simulink model "SkywalkerX8_StateEstimation"  (R2018a)
settings: Solver=FixedStepAuto  StartTime=0.0  StopTime=120  FixedStep=0.001  RelTol=1e-3
undefined symbols (not defined in the file): magnitude, SkywalkerX8
libraries: simulink_extras x10, sensors x7, sharedTrackingLibrary x2, dspmtrx3 x1
settings Model: Creator=David  LastModifiedBy=David

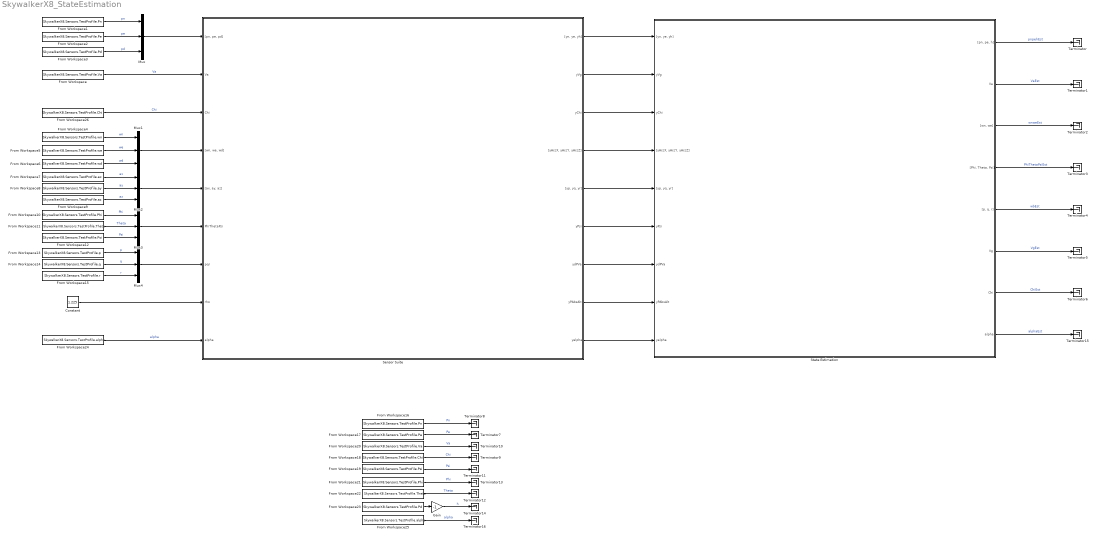
== system SkywalkerX8_StateEstimation ==
  Constant : Constant  Value=1.225
  From Workspace : FromWorkspace  VariableName=SkywalkerX8.Sensors.TestProfile.Va  SampleTime=SkywalkerX8.Sensors.TestProfile.Time(2)  Interpolate=off  OutputAfterFinalValue=Holding final value
  From Workspace1 : FromWorkspace  VariableName=SkywalkerX8.Sensors.TestProfile.Pn  SampleTime=SkywalkerX8.Sensors.TestProfile.Time(2)  Interpolate=off  OutputAfterFinalValue=Holding final value
  From Workspace10 : FromWorkspace  VariableName=SkywalkerX8.Sensors.TestProfile.Phi  SampleTime=SkywalkerX8.Sensors.TestProfile.Time(2)  Interpolate=off  OutputAfterFinalValue=Holding final value
  From Workspace11 : FromWorkspace  VariableName=SkywalkerX8.Sensors.TestProfile.Theta  SampleTime=SkywalkerX8.Sensors.TestProfile.Time(2)  Interpolate=off  OutputAfterFinalValue=Holding final value
  From Workspace12 : FromWorkspace  VariableName=SkywalkerX8.Sensors.TestProfile.Psi  SampleTime=SkywalkerX8.Sensors.TestProfile.Time(2)  Interpolate=off  OutputAfterFinalValue=Holding final value
  From Workspace13 : FromWorkspace  VariableName=SkywalkerX8.Sensors.TestProfile.p  SampleTime=SkywalkerX8.Sensors.TestProfile.Time(2)  Interpolate=off  OutputAfterFinalValue=Holding final value
  From Workspace14 : FromWorkspace  VariableName=SkywalkerX8.Sensors.TestProfile.q  SampleTime=SkywalkerX8.Sensors.TestProfile.Time(2)  Interpolate=off  OutputAfterFinalValue=Holding final value
  From Workspace15 : FromWorkspace  VariableName=SkywalkerX8.Sensors.TestProfile.r  SampleTime=SkywalkerX8.Sensors.TestProfile.Time(2)  Interpolate=off  OutputAfterFinalValue=Holding final value
  From Workspace16 : FromWorkspace  VariableName=SkywalkerX8.Sensors.TestProfile.Pn  Interpolate=off  OutputAfterFinalValue=Holding final value
  From Workspace17 : FromWorkspace  VariableName=SkywalkerX8.Sensors.TestProfile.Pe  Interpolate=off  OutputAfterFinalValue=Holding final value
  From Workspace18 : FromWorkspace  VariableName=SkywalkerX8.Sensors.TestProfile.Chi  Interpolate=off  OutputAfterFinalValue=Holding final value
  From Workspace19 : FromWorkspace  VariableName=SkywalkerX8.Sensors.TestProfile.Psi  Interpolate=off  OutputAfterFinalValue=Holding final value
  From Workspace2 : FromWorkspace  VariableName=SkywalkerX8.Sensors.TestProfile.Pe  SampleTime=SkywalkerX8.Sensors.TestProfile.Time(2)  Interpolate=off  OutputAfterFinalValue=Holding final value
  From Workspace20 : FromWorkspace  VariableName=SkywalkerX8.Sensors.TestProfile.Va  Interpolate=off  OutputAfterFinalValue=Holding final value
  From Workspace21 : FromWorkspace  VariableName=SkywalkerX8.Sensors.TestProfile.Phi  Interpolate=off  OutputAfterFinalValue=Holding final value
  From Workspace22 : FromWorkspace  VariableName=SkywalkerX8.Sensors.TestProfile.Theta  Interpolate=off  OutputAfterFinalValue=Holding final value
  From Workspace23 : FromWorkspace  VariableName=SkywalkerX8.Sensors.TestProfile.Pd  SampleTime=SkywalkerX8.Sensors.TestProfile.Time(2)  Interpolate=off  OutputAfterFinalValue=Holding final value
  From Workspace24 : FromWorkspace  VariableName=SkywalkerX8.Sensors.TestProfile.alpha  SampleTime=SkywalkerX8.Sensors.TestProfile.Time(2)  Interpolate=off  OutputAfterFinalValue=Holding final value
  From Workspace25 : FromWorkspace  VariableName=SkywalkerX8.Sensors.TestProfile.alpha  SampleTime=SkywalkerX8.Sensors.TestProfile.Time(2)  Interpolate=off  OutputAfterFinalValue=Holding final value
  From Workspace26 : FromWorkspace  VariableName=SkywalkerX8.Sensors.TestProfile.Chi  SampleTime=SkywalkerX8.Sensors.TestProfile.Time(2)  Interpolate=off  OutputAfterFinalValue=Holding final value
  From Workspace3 : FromWorkspace  VariableName=SkywalkerX8.Sensors.TestProfile.Pd  SampleTime=SkywalkerX8.Sensors.TestProfile.Time(2)  Interpolate=off  OutputAfterFinalValue=Holding final value
  From Workspace4 : FromWorkspace  VariableName=SkywalkerX8.Sensors.TestProfile.wn  SampleTime=SkywalkerX8.Sensors.TestProfile.Time(2)  Interpolate=off  OutputAfterFinalValue=Holding final value
  From Workspace5 : FromWorkspace  VariableName=SkywalkerX8.Sensors.TestProfile.we  SampleTime=SkywalkerX8.Sensors.TestProfile.Time(2)  Interpolate=off  OutputAfterFinalValue=Holding final value
  From Workspace6 : FromWorkspace  VariableName=SkywalkerX8.Sensors.TestProfile.wd  SampleTime=SkywalkerX8.Sensors.TestProfile.Time(2)  Interpolate=off  OutputAfterFinalValue=Holding final value
  From Workspace7 : FromWorkspace  VariableName=SkywalkerX8.Sensors.TestProfile.ax  SampleTime=SkywalkerX8.Sensors.TestProfile.Time(2)  Interpolate=off  OutputAfterFinalValue=Holding final value
  From Workspace8 : FromWorkspace  VariableName=SkywalkerX8.Sensors.TestProfile.ay  SampleTime=SkywalkerX8.Sensors.TestProfile.Time(2)  Interpolate=off  OutputAfterFinalValue=Holding final value
  From Workspace9 : FromWorkspace  VariableName=SkywalkerX8.Sensors.TestProfile.az  SampleTime=SkywalkerX8.Sensors.TestProfile.Time(2)  Interpolate=off  OutputAfterFinalValue=Holding final value
  Gain : Gain  Gain=-1
  Mux{,1..4} (5 alike) : Mux  Inputs=3
  Sensor Suite : Subsystem
      mask Display:
      | image('telemetry.jpg')
      | 
      | color('cyan')
      | 
      | port_label('input', 1, '[p_N, p_E, p_D] (m)', 'texMode', 'On')
      | port_label('input', 2, 'V_a (m/s)', 'texMode', 'On')
      | port_label('input', 3, '\chi (rad)', 'texMode', 'On')
      | port_label('input', 4, '[w_N, w_E, w_D] (m/s)', 'texMode', 'On')
      | port_label('input', 5, '{\bfa_{inertial}} (m/s^2)', 'texMode', 'on')
      | port_label('input', 6, '[\phi, \theta, \psi] (rad)', 'texMode', 'on')
      | port_label('input', 7, '{\bf\omega_b} (rad/s)', 'texMode', 'on')
      | port_label('input', 8, '\rho (kg/m^3)', 'texMode', 'on')
      | port_label('input', 9, '\alpha (rad)', 'texMode', 'on')
      | 
      | port_label('output', 1, '[y_{GPS_N}, y_{GPS_E}, y_{GPS_h}] (m)', 'texMode', 'On')
      | port_label('output', 2, 'y_{GPS_{Vg}} (m/s)', 'texMode', 'On')
      | port_label('output', 3, 'y_{GPS_{\chi}} (rad)', 'texMode', 'On')
      | port_label('output', 4, '[y_{accel_x}, y_{accel_y}, y_{accel_z}] (m/s^2)', 'texMode', 'on')
      | port_label('output', 5, '[y_p, y_q, y_r] (rad/s)', 'texMode', 'on')
      | port_label('output', 6, 'y_{\psi} (rad)', 'texMode', 'on')
      | port_label('output', 7, 'y_{\DeltaP_{V_a}} (Pa)', 'texMode', 'on')
      | port_label('output', 8, 'y_{P_{abs}} (Pa)', 'texMode', 'on')
      | port_label('output', 9, 'y_\alpha (rad)', 'texMode', 'on')
  State Estimation : Subsystem
      mask Display:
      | image('state_estimate.jpg', 'center')
      | 
      | port_label('input', 1, '[y_{GPS_N}, y_{GPS_E}, y_{GPS_h}] (m)', 'texMode', 'On')
      | port_label('input', 2, 'y_{GPS_{Vg}} (m/s)', 'texMode', 'On')
      | port_label('input', 3, 'y_{GPS_{\chi}} (rad)', 'texMode', 'On')
      | port_label('input', 4, '[y_{accel_x}, y_{accel_y}, y_{accel_z}] (m/s^2)', 'texMode', 'on')
      | port_label('input', 5, '[y_p, y_q, y_r] (rad/s)', 'texMode', 'on')
      | port_label('input', 6, 'y_{\psi} (rad)', 'texMode', 'on')
      | port_label('input', 7, 'y_{\DeltaP_{V_a}} (Pa)', 'texMode', 'on')
      | port_label('input', 8, 'y_{P_{abs}} (Pa)', 'texMode', 'on')
      | port_label('input', 9, 'y_{\alpha} (rad)', 'texMode', 'on')
      | 
      | port_label('output', 1, '[p_N, p_E, h] (m)', 'texMode', 'On')
      | port_label('output', 2, 'V_a (m/s)', 'texMode', 'On')
      | port_label('output', 3, '[w_N, w_E] (m/s)', 'texMode', 'On')
      | port_label('output', 4, '[\phi, \theta, \psi] (rad)', 'texMode', 'on')
      | port_label('output', 5, '{\bf\omega_b} (rad/s)', 'texMode', 'on')
      | port_label('output', 6, 'V_g (m/s)', 'texMode', 'on')
      | port_label('output', 7, '\chi (rad)', 'texMode', 'on')
      | port_label('output', 8, '\alpha (rad)', 'texMode', 'on')
  Terminator{,1..16} (17 alike) : Terminator
  wires:
  Mux2/1 -> Sensor Suite/5("[ax, ay, az]")
  From Workspace14/1 -> Mux4/2  "q"
  From Workspace2/1 -> Mux/2  "pe"
  From Workspace10/1 -> Mux3/1  "Phi"
  Mux1/1 -> Sensor Suite/4("[wn, we, wd]")
  From Workspace13/1 -> Mux4/1  "p"
  From Workspace1/1 -> Mux/1  "pn"
  Constant/1 -> Sensor Suite/8(rho)
  From Workspace11/1 -> Mux3/2  "Theta"
  From Workspace4/1 -> Mux1/1  "wn"
  From Workspace7/1 -> Mux2/1  "ax"
  From Workspace6/1 -> Mux1/3  "wd"
  From Workspace9/1 -> Mux2/3  "az"
  From Workspace12/1 -> Mux3/3  "Psi"
  From Workspace/1 -> Sensor Suite/2(Va)  "Va"
  From Workspace3/1 -> Mux/3  "pd"
  Mux4/1 -> Sensor Suite/7(pqr)
  From Workspace8/1 -> Mux2/2  "ay"
  Mux3/1 -> Sensor Suite/6(PhiThetaPsi)
  From Workspace5/1 -> Mux1/2  "we"
  From Workspace15/1 -> Mux4/3  "r"
  Mux/1 -> Sensor Suite/1("[pn, pe, pd]")
  State Estimation/1("[pn, pe, h]") -> Terminator/1  "pnpehEst"
  State Estimation/2(Va) -> Terminator1/1  "VaEst"
  State Estimation/3("[wn, we]") -> Terminator2/1  "wnweEst"
  State Estimation/4("[Phi, Theta, Psi]") -> Terminator3/1  "PhiThetaPsiEst"
  State Estimation/5("[p, q, r]") -> Terminator4/1  "wbEst"
  State Estimation/6(Vg) -> Terminator5/1  "VgEst"
  State Estimation/7(Chi) -> Terminator6/1  "ChiEst"
  From Workspace20/1 -> Terminator10/1  "Va"
  From Workspace16/1 -> Terminator8/1  "Pn"
  From Workspace18/1 -> Terminator9/1  "Chi"
  From Workspace19/1 -> Terminator11/1  "Psi"
  From Workspace17/1 -> Terminator7/1  "Pe"
  From Workspace21/1 -> Terminator13/1  "Phi"
  From Workspace22/1 -> Terminator12/1  "Theta"
  From Workspace23/1 -> Gain/1
  Gain/1 -> Terminator14/1  "h"
  Sensor Suite/9(yalpha) -> State Estimation/9(yalpha)
  Sensor Suite/8(yPAbsAlt) -> State Estimation/8(yPAbsAlt)
  Sensor Suite/7(ydPVa) -> State Estimation/7(ydPVa)
  Sensor Suite/6(yPsi) -> State Estimation/6(yPsi)
  Sensor Suite/5("[yp, yq, yr]") -> State Estimation/5("[yp, yq, yr]")
  Sensor Suite/4("[yAccX, yAccY, yAccZ]") -> State Estimation/4("[yAccX, yAccY, yAccZ]")
  Sensor Suite/3(yChi) -> State Estimation/3(yChi)
  Sensor Suite/2(yVg) -> State Estimation/2(yVg)
  Sensor Suite/1("[yn, ye, yh]") -> State Estimation/1("[yn, ye, yh]")
  State Estimation/8(alpha) -> Terminator15/1  "alphaEst"
  From Workspace24/1 -> Sensor Suite/9(alpha)  "alpha"
  From Workspace25/1 -> Terminator16/1  "alpha"
  From Workspace26/1 -> Sensor Suite/3(Chi)  "Chi"

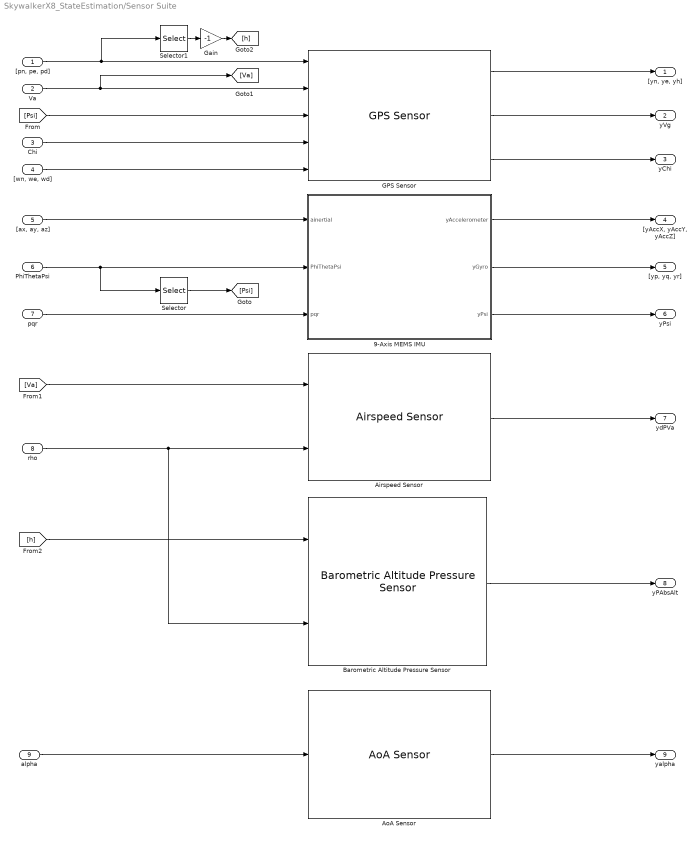
== system SkywalkerX8_StateEstimation/Sensor Suite ==
  "[pn, pe, pd]" : Inport
  Va : Inport  Port=2
  Chi : Inport  Port=3
  "[wn, we, wd]" : Inport  Port=4
  "[ax, ay, az]" : Inport  Port=5
  PhiThetaPsi : Inport  Port=6
  pqr : Inport  Port=7
  rho : Inport  Port=8
  alpha : Inport  Port=9
  9-Axis MEMS IMU : Subsystem
      mask Display:
      | image('VNAV_IMU.jpg')
      | 
      | color('green')
      | 
      | port_label('input', 1, '{\bfa_{inertial}} (m/s^2)', 'texMode', 'on')
      | port_label('input', 2, '[\phi, \theta, \psi] (rad)', 'texMode', 'on')
      | port_label('input', 3, '{\bf\omega_b} (rad/s)', 'texMode', 'on')
      | 
      | port_label('output', 1, '[y_{accel_x}, y_{accel_y}, y_{accel_z}] (m/s^2)', 'texMode', 'on')
      | port_label('output', 2, '[y_p, y_q, y_r] (rad/s)', 'texMode', 'on')
      | port_label('output', 3, 'y_{\psi} (rad)', 'texMode', 'on')
  Airspeed Sensor : sensors/Airspeed Sensor  SampleTime=SkywalkerX8.Sensors.AirspeedPressure.SampleTime  diffPressureStdDev=SkywalkerX8.Sensors.AirspeedPressure.StdDev  diffPressureBandwidthHz=SkywalkerX8.Sensors.AirspeedPressure.BandwidthHz  diffPressureInit=SkywalkerX8.Sensors.AirspeedPressure.InitialCondition  diffPressureUpperSaturation=SkywalkerX8.Sensors.AirspeedPressure.UpperSat  diffPressureLowerSaturation=SkywalkerX8.Sensors.AirspeedPressure.LowerSat  diffPressureResolution=SkywalkerX8.Sensors.AirspeedPressure.Resolution
  AoA Sensor : sensors/AoA Sensor  SampleTime=SkywalkerX8.Sensors.AoA.SampleTime  alphaStdDev=SkywalkerX8.Sensors.AoA.StdDev  alphaBandwidthHz=SkywalkerX8.Sensors.AoA.BandwidthHz  alphaInit=SkywalkerX8.Sensors.AoA.InitialCondition  alphaUpperSaturation=SkywalkerX8.Sensors.AoA.UpperSat  alphaLowerSaturation=SkywalkerX8.Sensors.AoA.LowerSat  alphaResolution=SkywalkerX8.Sensors.AoA.Resolution
  Barometric Altitude Pressure Sensor : sensors/Barometric Altitude Pressure Sensor  g=SkywalkerX8.System.Gravity  SampleTime=SkywalkerX8.Sensors.AltitudePressure.SampleTime  absPressureStdDev=SkywalkerX8.Sensors.AltitudePressure.StdDev  absPressureBandwidthHz=SkywalkerX8.Sensors.AltitudePressure.BandwidthHz  absPressureInit=SkywalkerX8.Sensors.AltitudePressure.InitialCondition  absPressureUpperSaturation=SkywalkerX8.Sensors.AltitudePressure.UpperSat  absPressureLowerSaturation=SkywalkerX8.Sensors.AltitudePressure.LowerSat  absPressureResolution=SkywalkerX8.Sensors.AltitudePressure.Resolution
  GPS Sensor : sensors/GPS Sensor  SampleTime=SkywalkerX8.Sensors.GPS.SampleTime  pnInit=SkywalkerX8.Sensors.GPS.pnInit  peInit=SkywalkerX8.Sensors.GPS.peInit  pdInit=SkywalkerX8.Sensors.GPS.pdInit  VgInit=SkywalkerX8.Sensors.GPS.VgInit  ChiInit=SkywalkerX8.Sensors.GPS.ChiInit  GPSNStdDev=SkywalkerX8.Sensors.GPS.North.StdDev  OneOverkGPSN=SkywalkerX8.Sensors.GPS.North.TimeConstant  GPSEStdDev=SkywalkerX8.Sensors.GPS.East.StdDev  OneOverkGPSE=SkywalkerX8.Sensors.GPS.East.TimeConstant  GPSAltStdDev=SkywalkerX8.Sensors.GPS.Alt.StdDev  OneOverkGPSAlt=SkywalkerX8.Sensors.GPS.Alt.TimeConstant  GPSVStdDev=SkywalkerX8.Sensors.GPS.Velocity.StdDev
  Gain : Gain  Gain=-1
  Selector : Selector  InputPortWidth=3  IndexOptions=Index vector (dialog)  Indices=3  OutputSizes=1
  Selector1 : Selector  InputPortWidth=3  IndexOptions=Index vector (dialog)  Indices=3  OutputSizes=1
  "[yn, ye, yh]" : Outport
  yVg : Outport  Port=2
  yChi : Outport  Port=3
  "[yAccX, yAccY, yAccZ]" : Outport  Port=4
  "[yp, yq, yr]" : Outport  Port=5
  yPsi : Outport  Port=6
  ydPVa : Outport  Port=7
  yPAbsAlt : Outport  Port=8
  yalpha : Outport  Port=9
  wires:
  "[pn, pe, pd]"/1 -> GPS Sensor/1, Selector1/1
  Va/1 -> GPS Sensor/2, [Va]
  PhiThetaPsi/1 -> 9-Axis MEMS IMU/2(PhiThetaPsi), Selector/1
  Airspeed Sensor/1 -> ydPVa/1
  [Psi] -> GPS Sensor/3
  Selector1/1 -> Gain/1
  rho/1 -> Barometric Altitude Pressure Sensor/2, Airspeed Sensor/2
  GPS Sensor/3 -> yChi/1
  Selector/1 -> [Psi]
  [h] -> Barometric Altitude Pressure Sensor/1
  9-Axis MEMS IMU/3(yPsi) -> yPsi/1
  [Va] -> Airspeed Sensor/1
  pqr/1 -> 9-Axis MEMS IMU/3(pqr)
  9-Axis MEMS IMU/2(yGyro) -> "[yp, yq, yr]"/1
  "[wn, we, wd]"/1 -> GPS Sensor/5
  Barometric Altitude Pressure Sensor/1 -> yPAbsAlt/1
  GPS Sensor/1 -> "[yn, ye, yh]"/1
  Gain/1 -> [h]
  GPS Sensor/2 -> yVg/1
  "[ax, ay, az]"/1 -> 9-Axis MEMS IMU/1(ainertial)
  9-Axis MEMS IMU/1(yAccelerometer) -> "[yAccX, yAccY, yAccZ]"/1
  AoA Sensor/1 -> yalpha/1
  alpha/1 -> AoA Sensor/1
  Chi/1 -> GPS Sensor/4

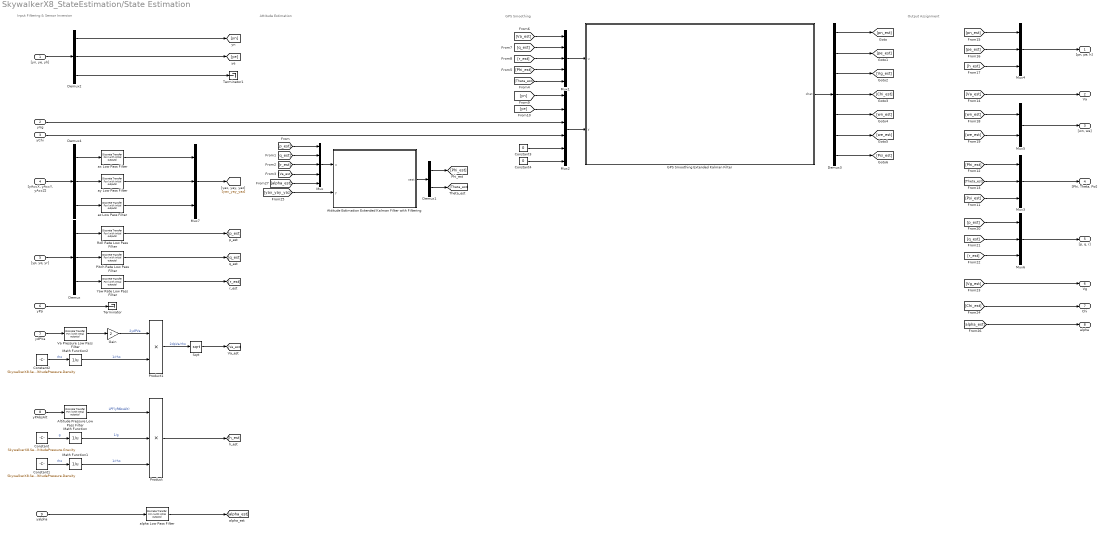
== system SkywalkerX8_StateEstimation/State Estimation ==
  note: Output Assignment
  note: GPS Smoothing
  note: Attitude Estimation
  note: Input Filtering & Sensor Inversion
  "[yn, ye, yh]" : Inport  PortDimensions=3
  yVg : Inport  Port=2
  yChi : Inport  Port=3
  "[yAccX, yAccY, yAccZ]" : Inport  Port=4  PortDimensions=3
  "[yp, yq, yr]" : Inport  Port=5  PortDimensions=3
  yPsi : Inport  Port=6
  ydPVa : Inport  Port=7
  yPAbsAlt : Inport  Port=8
  yalpha : Inport  Port=9
  Altitude Pressure Low Pass Filter : simulink_extras/Additional Discrete/Discrete Transfer Fcn (with initial outputs)  N=cell2mat(SkywalkerX8.Sensors.Filters.AltitudePressure.FilterTFDigital.Numerator)  D=cell2mat(SkywalkerX8.Sensors.Filters.AltitudePressure.FilterTFDigital.Denominator)  U0=SkywalkerX8.Sensors.Filters.AltitudePressure.InitialCondition  Y0=SkywalkerX8.Sensors.Filters.AltitudePressure.InitialCondition  TS=SkywalkerX8.Sensors.Filters.AltitudePressure.FilterSampleTime
      settings: SourceProductName=Simulink  SourceProductBaseCode=SL
  Attitude Estimation Extended Kalman Filter with Filtering : Subsystem
      mask Display:
      | port_label('input', 1, '{\bf u} = [p, q, r, V_a, \alpha]', 'texMode', 'On')
      | port_label('input', 2, '{\bf y} = [a_x, a_y, a_z]', 'texMode', 'On')
      | 
      | port_label('output', 1, '{\bf x_{est}} = [\Phi, \theta]', 'texMode', 'On')
  Constant : Constant  Value=SkywalkerX8.Sensors.StateEstimate.SensorInversion.AltitudePressure.Gravity
  Constant1 : Constant  Value=SkywalkerX8.Sensors.StateEstimate.SensorInversion.AltitudePressure.Density
  Constant2 : Constant  Value=SkywalkerX8.Sensors.StateEstimate.SensorInversion.AltitudePressure.Density
  Constant3 : Constant  Value=0
  Constant4 : Constant  Value=0
  Demux : Demux  Outputs=3
  Demux1 : Demux  Outputs=2
  Demux2 : Demux  Outputs=3
  Demux3 : Demux  Outputs=7
  Demux4 : Demux  Outputs=3
  GPS Smoothing Extended Kalman Filter : Subsystem
      mask Display:
      | port_label('input', 1, '{\bf u} = [V_a, q, r, \Phi, \theta]', 'texMode', 'On')
      | port_label('input', 2, '{\bf y} = [y_{GPS_N}, y_{GPS_E}, y_{GPS_{V_g}}, y_{GPS_\chi}, y_{GPS_{wind_N}}, y_{GPS_{wind_E}}]', 'texMode', 'On')
      | 
      | port_label('output', 1, '{\bf x_{est}} = [p_n, p_e, V_g, \chi, w_n, w_e, \psi]', 'texMode', 'On')
  Gain : Gain  Gain=2
  Math Function : Math  Operator=reciprocal  SaturateOnIntegerOverflow=on
  Math Function1 : Math  Operator=reciprocal  SaturateOnIntegerOverflow=on
  Math Function2 : Math  Operator=reciprocal  SaturateOnIntegerOverflow=on
  Mux : Mux  Inputs=5
  Mux1 : Mux  Inputs=5
  Mux2 : Mux  Inputs=6
  Mux{3..4,6..7} (4 alike) : Mux  Inputs=3
  Mux5 : Mux  Inputs=2
  Pitch Rate Low Pass Filter : simulink_extras/Additional Discrete/Discrete Transfer Fcn (with initial outputs)  N=cell2mat(SkywalkerX8.Sensors.Filters.AngularRates.Pitch.FilterTFDigital.Numerator)  D=cell2mat(SkywalkerX8.Sensors.Filters.AngularRates.Pitch.FilterTFDigital.Denominator)  U0=SkywalkerX8.Sensors.Filters.AngularRates.Pitch.InitialCondition  Y0=SkywalkerX8.Sensors.Filters.AngularRates.Pitch.InitialCondition  TS=SkywalkerX8.Sensors.Filters.AngularRates.Pitch.FilterSampleTime
      settings: SourceProductName=Simulink  SourceProductBaseCode=SL
  Product : Product  Inputs=3
  Product1 : Product
  Roll Rate Low Pass Filter : simulink_extras/Additional Discrete/Discrete Transfer Fcn (with initial outputs)  N=cell2mat(SkywalkerX8.Sensors.Filters.AngularRates.Roll.FilterTFDigital.Numerator)  D=cell2mat(SkywalkerX8.Sensors.Filters.AngularRates.Roll.FilterTFDigital.Denominator)  U0=SkywalkerX8.Sensors.Filters.AngularRates.Roll.InitialCondition  Y0=SkywalkerX8.Sensors.Filters.AngularRates.Roll.InitialCondition  TS=SkywalkerX8.Sensors.Filters.AngularRates.Roll.FilterSampleTime
      settings: SourceProductName=Simulink  SourceProductBaseCode=SL
  Sqrt : Sqrt  SaturateOnIntegerOverflow=on
  Terminator : Terminator
  Terminator1 : Terminator
  Va Pressure Low Pass Filter : simulink_extras/Additional Discrete/Discrete Transfer Fcn (with initial outputs)  N=cell2mat(SkywalkerX8.Sensors.Filters.AirspeedPressure.FilterTFDigital.Numerator)  D=cell2mat(SkywalkerX8.Sensors.Filters.AirspeedPressure.FilterTFDigital.Denominator)  U0=SkywalkerX8.Sensors.Filters.AirspeedPressure.InitialCondition  Y0=SkywalkerX8.Sensors.Filters.AirspeedPressure.InitialCondition  TS=SkywalkerX8.Sensors.Filters.AirspeedPressure.FilterSampleTime
      settings: SourceProductName=Simulink  SourceProductBaseCode=SL
  Yaw Rate Low Pass Filter : simulink_extras/Additional Discrete/Discrete Transfer Fcn (with initial outputs)  N=cell2mat(SkywalkerX8.Sensors.Filters.AngularRates.Yaw.FilterTFDigital.Numerator)  D=cell2mat(SkywalkerX8.Sensors.Filters.AngularRates.Yaw.FilterTFDigital.Denominator)  U0=SkywalkerX8.Sensors.Filters.AngularRates.Yaw.InitialCondition  Y0=SkywalkerX8.Sensors.Filters.AngularRates.Yaw.InitialCondition  TS=SkywalkerX8.Sensors.Filters.AngularRates.Yaw.FilterSampleTime
      settings: SourceProductName=Simulink  SourceProductBaseCode=SL
  alpha Low Pass Filter : simulink_extras/Additional Discrete/Discrete Transfer Fcn (with initial outputs)  N=cell2mat(SkywalkerX8.Sensors.Filters.AoA.FilterTFDigital.Numerator)  D=cell2mat(SkywalkerX8.Sensors.Filters.AoA.FilterTFDigital.Denominator)  U0=SkywalkerX8.Sensors.Filters.AoA.InitialCondition  Y0=SkywalkerX8.Sensors.Filters.AoA.InitialCondition  TS=SkywalkerX8.Sensors.Filters.AoA.FilterSampleTime
      settings: SourceProductName=Simulink  SourceProductBaseCode=SL
  ax Low Pass Filter : simulink_extras/Additional Discrete/Discrete Transfer Fcn (with initial outputs)  N=cell2mat(SkywalkerX8.Sensors.EKF.Attitude.Filters.axFilterTFDigital.Numerator)  D=cell2mat(SkywalkerX8.Sensors.EKF.Attitude.Filters.axFilterTFDigital.Denominator)  U0=SkywalkerX8.Sensors.EKF.Attitude.InitialMeasurement(1)  Y0=SkywalkerX8.Sensors.EKF.Attitude.InitialMeasurement(1)  TS=SkywalkerX8.Sensors.EKF.Attitude.Filters.aFilterSampleTime
      settings: SourceProductName=Simulink  SourceProductBaseCode=SL
  ay Low Pass Filter : simulink_extras/Additional Discrete/Discrete Transfer Fcn (with initial outputs)  N=cell2mat(SkywalkerX8.Sensors.EKF.Attitude.Filters.ayFilterTFDigital.Numerator)  D=cell2mat(SkywalkerX8.Sensors.EKF.Attitude.Filters.ayFilterTFDigital.Denominator)  U0=SkywalkerX8.Sensors.EKF.Attitude.InitialMeasurement(2)  Y0=SkywalkerX8.Sensors.EKF.Attitude.InitialMeasurement(2)  TS=SkywalkerX8.Sensors.EKF.Attitude.Filters.aFilterSampleTime
      settings: SourceProductName=Simulink  SourceProductBaseCode=SL
  az Low Pass Filter : simulink_extras/Additional Discrete/Discrete Transfer Fcn (with initial outputs)  N=cell2mat(SkywalkerX8.Sensors.EKF.Attitude.Filters.azFilterTFDigital.Numerator)  D=cell2mat(SkywalkerX8.Sensors.EKF.Attitude.Filters.azFilterTFDigital.Denominator)  U0=SkywalkerX8.Sensors.EKF.Attitude.InitialMeasurement(3)  Y0=SkywalkerX8.Sensors.EKF.Attitude.InitialMeasurement(3)  TS=SkywalkerX8.Sensors.EKF.Attitude.Filters.aFilterSampleTime
      settings: SourceProductName=Simulink  SourceProductBaseCode=SL
  "[pn, pe, h]" : Outport
  Va : Outport  Port=2
  "[wn, we]" : Outport  Port=3
  "[Phi, Theta, Psi]" : Outport  Port=4
  "[p, q, r]" : Outport  Port=5
  Vg : Outport  Port=6
  Chi : Outport  Port=7
  alpha : Outport  Port=8
  wires:
  [Phi_est] -> Mux1/4
  Math Function1/1 -> Product/3  "1/rho"
  [ye] -> Mux2/2
  Sqrt/1 -> [Va_est]
  Demux/2 -> Pitch Rate Low Pass Filter/1
  [r_est] -> Mux/3
  Math Function2/1 -> Product1/2  "1/rho"
  yChi/1 -> Mux2/4
  Demux2/3 -> Terminator1/1
  Mux4/1 -> "[pn, pe, h]"/1
  Mux6/1 -> "[p, q, r]"/1
  [r_est] -> Mux1/3
  Constant3/1 -> Mux2/5
  Constant2/1 -> Math Function2/1  "rho"
  Demux3/4 -> [Chi_est]
  Demux3/3 -> [Vg_est]
  [h_est] -> Mux4/3
  Math Function/1 -> Product/2  "1/g"
  [we_est] -> Mux5/2
  "[yp, yq, yr]"/1 -> Demux/1
  [Theta_est] -> Mux1/5
  Demux3/7 -> [Psi_est]
  Mux2/1 -> GPS Smoothing Extended Kalman Filter/2(y)
  Constant4/1 -> Mux2/6
  [r_est] -> Mux6/3
  Mux/1 -> Attitude Estimation Extended Kalman Filter with Filtering/1(u)
  [wn_est] -> Mux5/1
  Demux2/2 -> [ye]
  GPS Smoothing Extended Kalman Filter/1(xhat) -> Demux3/1
  Constant1/1 -> Math Function1/1  "rho"
  Demux2/1 -> [yn]
  Demux3/6 -> [we_est]
  [q_est] -> Mux6/2
  "[yAccX, yAccY, yAccZ]"/1 -> Demux4/1
  Demux1/2 -> [Theta_est]
  Mux1/1 -> GPS Smoothing Extended Kalman Filter/1(u)
  Demux3/5 -> [wn_est]
  Attitude Estimation Extended Kalman Filter with Filtering/1(xest) -> Demux1/1
  Gain/1 -> Product1/1  "2ydPVa"
  Constant/1 -> Math Function/1  "g"
  [p_est] -> Mux/1
  yVg/1 -> Mux2/3
  Altitude Pressure Low Pass Filter/1 -> Product/1  "LPF(yPAbsAlt)"
  [Chi_est] -> Chi/1
  yPsi/1 -> Terminator/1
  [q_est] -> Mux1/2
  Demux3/1 -> [pn_est]
  [Va_est] -> Mux1/1
  [Theta_est] -> Mux3/2
  Va Pressure Low Pass Filter/1 -> Gain/1
  [q_est] -> Mux/2
  Product1/1 -> Sqrt/1  "2dpVa/rho"
  Yaw Rate Low Pass Filter/1 -> [r_est]
  Product/1 -> [h_est]
  [Va_est] -> Mux/4
  ydPVa/1 -> Va Pressure Low Pass Filter/1
  [Psi_est] -> Mux3/3
  Pitch Rate Low Pass Filter/1 -> [q_est]
  Demux/1 -> Roll Rate Low Pass Filter/1
  yPAbsAlt/1 -> Altitude Pressure Low Pass Filter/1
  Demux/3 -> Yaw Rate Low Pass Filter/1
  [pn_est] -> Mux4/1
  [p_est] -> Mux6/1
  Demux3/2 -> [pe_est]
  Demux1/1 -> [Phi_est]
  [Vg_est] -> Vg/1
  "[yn, ye, yh]"/1 -> Demux2/1
  [pe_est] -> Mux4/2
  [Phi_est] -> Mux3/1
  Mux3/1 -> "[Phi, Theta, Psi]"/1
  Mux5/1 -> "[wn, we]"/1
  [Va_est] -> Va/1
  [yn] -> Mux2/1
  Roll Rate Low Pass Filter/1 -> [p_est]
  Demux4/1 -> ax Low Pass Filter/1
  Demux4/2 -> ay Low Pass Filter/1
  Demux4/3 -> az Low Pass Filter/1
  ax Low Pass Filter/1 -> Mux7/1
  ay Low Pass Filter/1 -> Mux7/2
  az Low Pass Filter/1 -> Mux7/3
  Mux7/1 -> [yax_yay_yaz]
  [yax_yay_yaz] -> Attitude Estimation Extended Kalman Filter with Filtering/2(y)
  yalpha/1 -> alpha Low Pass Filter/1
  alpha Low Pass Filter/1 -> [alpha_est]
  [alpha_est] -> alpha/1
  [alpha_est] -> Mux/5

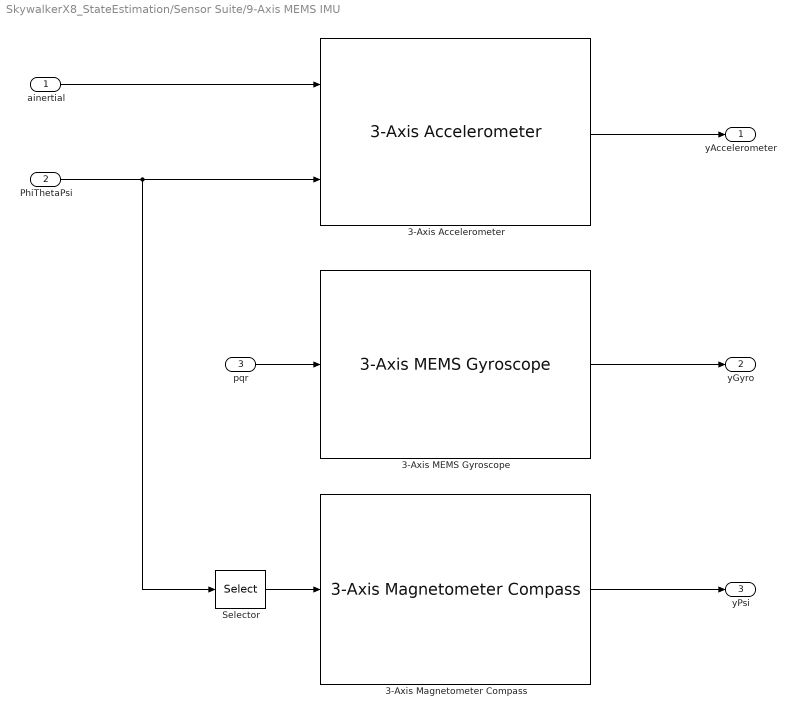
== system SkywalkerX8_StateEstimation/Sensor Suite/9-Axis MEMS IMU ==
  ainertial : Inport
  PhiThetaPsi : Inport  Port=2
  pqr : Inport  Port=3
  3-Axis Accelerometer : sensors/3-Axis Accelerometer  g=SkywalkerX8.System.Gravity  SampleTime=SkywalkerX8.Sensors.IMU.Accelerometer.SampleTime  accelXNoiseDensity=SkywalkerX8.Sensors.IMU.Accelerometer.X.NoiseDensity  accelYNoiseDensity=SkywalkerX8.Sensors.IMU.Accelerometer.Y.NoiseDensity  accelZNoiseDensity=SkywalkerX8.Sensors.IMU.Accelerometer.Z.NoiseDensity  accelXBandwidthHz=SkywalkerX8.Sensors.IMU.Accelerometer.X.BandwidthHz  accelYBandwidthHz=SkywalkerX8.Sensors.IMU.Accelerometer.Y.BandwidthHz  accelZBandwidthHz=SkywalkerX8.Sensors.IMU.Accelerometer.Z.BandwidthHz  accelXInit=SkywalkerX8.Sensors.IMU.Accelerometer.X.InitialCondition  accelYInit=SkywalkerX8.Sensors.IMU.Accelerometer.Y.InitialCondition  accelZInit=SkywalkerX8.Sensors.IMU.Accelerometer.Z.InitialCondition  accelXUpperSaturation=SkywalkerX8.Sensors.IMU.Accelerometer.X.UpperSat  accelXLowerSaturation=SkywalkerX8.Sensors.IMU.Accelerometer.X.LowerSat  accelYUpperSaturation=SkywalkerX8.Sensors.IMU.Accelerometer.Y.UpperSat  accelYLowerSaturation=SkywalkerX8.Sensors.IMU.Accelerometer.Y.LowerSat  accelZUpperSaturation=SkywalkerX8.Sensors.IMU.Accelerometer.Z.UpperSat  accelZLowerSaturation=SkywalkerX8.Sensors.IMU.Accelerometer.Z.LowerSat  accelXResolution=SkywalkerX8.Sensors.IMU.Accelerometer.X.Resolution  accelYResolution=SkywalkerX8.Sensors.IMU.Accelerometer.Y.Resolution  accelZResolution=SkywalkerX8.Sensors.IMU.Accelerometer.Z.Resolution
  3-Axis MEMS Gyroscope : sensors/3-Axis MEMS Gyroscope  SampleTime=SkywalkerX8.Sensors.IMU.Gyroscope.SampleTime  gyroXNoiseDensity=SkywalkerX8.Sensors.IMU.Gyroscope.X.NoiseDensity  gyroYNoiseDensity=SkywalkerX8.Sensors.IMU.Gyroscope.Y.NoiseDensity  gyroZNoiseDensity=SkywalkerX8.Sensors.IMU.Gyroscope.Z.NoiseDensity  gyroXBandwidthHz=SkywalkerX8.Sensors.IMU.Gyroscope.X.BandwidthHz  gyroYBandwidthHz=SkywalkerX8.Sensors.IMU.Gyroscope.Y.BandwidthHz  gyroZBandwidthHz=SkywalkerX8.Sensors.IMU.Gyroscope.Z.BandwidthHz  gyroXInit=SkywalkerX8.Sensors.IMU.Gyroscope.X.InitialCondition  gyroYInit=SkywalkerX8.Sensors.IMU.Gyroscope.Y.InitialCondition  gyroZInit=SkywalkerX8.Sensors.IMU.Gyroscope.Z.InitialCondition  gyroXUpperSaturation=SkywalkerX8.Sensors.IMU.Gyroscope.X.UpperSat  gyroXLowerSaturation=SkywalkerX8.Sensors.IMU.Gyroscope.X.LowerSat  gyroYUpperSaturation=SkywalkerX8.Sensors.IMU.Gyroscope.Y.UpperSat  gyroYLowerSaturation=SkywalkerX8.Sensors.IMU.Gyroscope.Y.LowerSat  gyroZUpperSaturation=SkywalkerX8.Sensors.IMU.Gyroscope.Z.UpperSat  gyroZLowerSaturation=SkywalkerX8.Sensors.IMU.Gyroscope.Z.LowerSat  gyroXResolution=SkywalkerX8.Sensors.IMU.Gyroscope.X.Resolution  gyroYResolution=SkywalkerX8.Sensors.IMU.Gyroscope.Y.Resolution  gyroZResolution=SkywalkerX8.Sensors.IMU.Gyroscope.Z.Resolution
  3-Axis Magnetometer Compass : sensors/3-Axis Magnetometer Compass  SampleTime=SkywalkerX8.Sensors.IMU.Compass.SampleTime  headingNoiseDensity=SkywalkerX8.Sensors.IMU.Compass.NoiseDensity  headingBandwidthHz=SkywalkerX8.Sensors.IMU.Compass.BandwidthHz  headingInit=SkywalkerX8.Sensors.IMU.Compass.InitialCondition  headingUpperSaturation=SkywalkerX8.Sensors.IMU.Compass.UpperSat  headingLowerSaturation=SkywalkerX8.Sensors.IMU.Compass.LowerSat  headingResolution=SkywalkerX8.Sensors.IMU.Compass.Resolution
  Selector : Selector  InputPortWidth=3  IndexOptions=Index vector (dialog)  Indices=3  OutputSizes=1
  yAccelerometer : Outport
  yGyro : Outport  Port=2
  yPsi : Outport  Port=3
  wires:
  ainertial/1 -> 3-Axis Accelerometer/1
  PhiThetaPsi/1 -> 3-Axis Accelerometer/2, Selector/1
  Selector/1 -> 3-Axis Magnetometer Compass/1
  pqr/1 -> 3-Axis MEMS Gyroscope/1
  3-Axis MEMS Gyroscope/1 -> yGyro/1
  3-Axis Accelerometer/1 -> yAccelerometer/1
  3-Axis Magnetometer Compass/1 -> yPsi/1

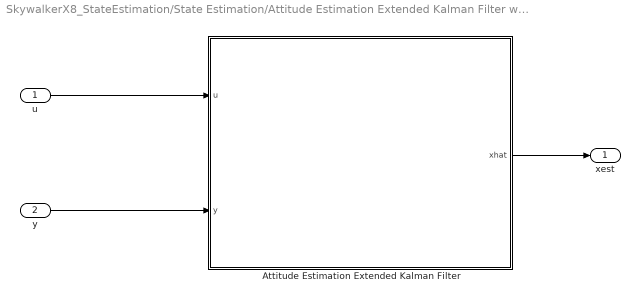
== system SkywalkerX8_StateEstimation/State Estimation/Attitude Estimation Extended Kalman Filter with Filtering ==
  u : Inport
  y : Inport  Port=2
  Attitude Estimation Extended Kalman Filter : Subsystem
      mask Display:
      | port_label('input', 1, '{\bf u} = [p, q, r, V_a, \alpha]', 'texMode', 'On')
      | port_label('input', 2, '{\bf y} = [a_x, a_y, a_z]', 'texMode', 'On')
      | 
      | port_label('output', 1, '{\bf x_{est}} = [\Phi, \theta]', 'texMode', 'On')
  xest : Outport
  wires:
  y/1 -> Attitude Estimation Extended Kalman Filter/2(y)
  Attitude Estimation Extended Kalman Filter/1(xhat) -> xest/1
  u/1 -> Attitude Estimation Extended Kalman Filter/1(u)

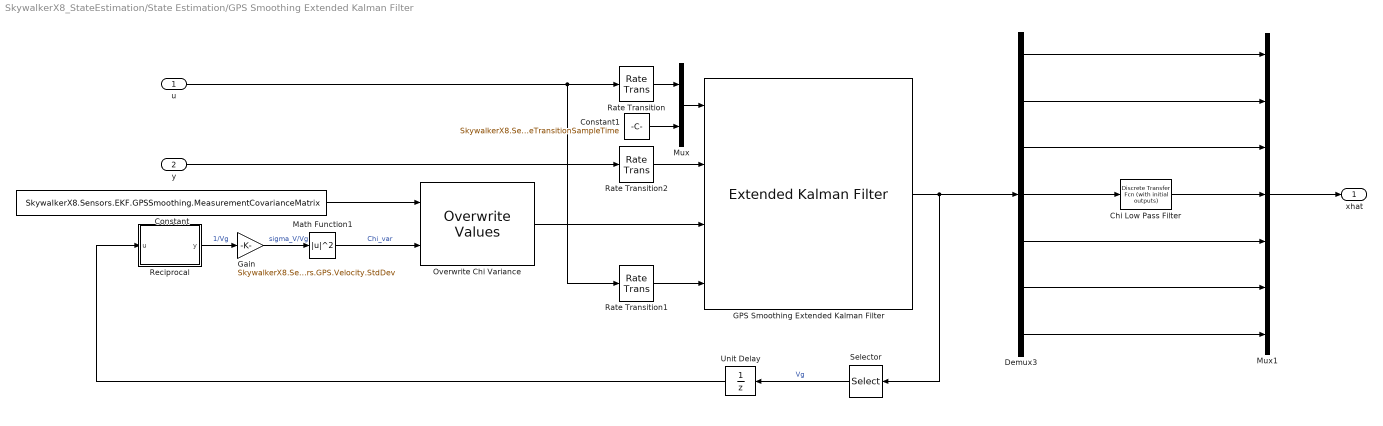
== system SkywalkerX8_StateEstimation/State Estimation/GPS Smoothing Extended Kalman Filter ==
  u : Inport  PortDimensions=5
  y : Inport  Port=2  PortDimensions=6
  Chi Low Pass Filter : simulink_extras/Additional Discrete/Discrete Transfer Fcn (with initial outputs)  N=cell2mat(SkywalkerX8.Sensors.EKF.GPSSmoothing.Filters.ChiFilter.TFDigital.Numerator)  D=cell2mat(SkywalkerX8.Sensors.EKF.GPSSmoothing.Filters.ChiFilter.TFDigital.Denominator)  U0=SkywalkerX8.Sensors.EKF.GPSSmoothing.Filters.ChiFilter.InitialCondition  Y0=SkywalkerX8.Sensors.EKF.GPSSmoothing.Filters.ChiFilter.InitialCondition  TS=SkywalkerX8.Sensors.EKF.GPSSmoothing.Filters.ChiFilter.SampleTime
      settings: SourceProductName=Simulink  SourceProductBaseCode=SL
  Constant : Constant  Value=SkywalkerX8.Sensors.EKF.GPSSmoothing.MeasurementCovarianceMatrix
  Constant1 : Constant  Value=SkywalkerX8.Sensors.EKF.GPSSmoothing.StateTransitionSampleTime
  Demux3 : Demux  Outputs=7
  GPS Smoothing Extended Kalman Filter : sharedTrackingLibrary/Extended Kalman Filter  StateTransitionFcn=GPSSmoothingTransitionEstimate  HasStateTransitionJacobianFcn=on  StateTransitionJacobianFcn=GPSSmoothingTransitionEstimate_Jacobian  HasAdditiveProcessNoise=Additive  ProcessNoise=SkywalkerX8.Sensors.EKF.GPSSmoothing.ProcessCovarianceMatrix  HasTimeVaryingProcessNoise=off  HasStateTransitionFcnExtraArgument=1  InitialState=SkywalkerX8.Sensors.EKF.GPSSmoothing.InitialState  InitialStateCovariance=SkywalkerX8.Sensors.EKF.GPSSmoothing.InitialStateCovarianceMatrix  MeasurementFcn1=GPSSmoothingMeasurementEstimate  HasMeasurementJacobianFcn1=on  MeasurementJacobianFcn1=GPSSmoothingMeasurementEstimate_Jacobian  HasMeasurementEnablePort1=off  HasAdditiveMeasurementNoise1=Additive  MeasurementNoise1=SkywalkerX8.Sensors.EKF.GPSSmoothing.MeasurementCovarianceMatrix  HasTimeVaryingMeasurementNoise1=on  HasMeasurementFcnExtraArgument1=1  MeasurementFcn2=myMeasurementFcn  HasMeasurementJacobianFcn2=off  HasMeasurementEnablePort2=off  HasAdditiveMeasurementNoise2=Additive  MeasurementNoise2=1  HasTimeVaryingMeasurementNoise2=off  HasMeasurementFcnExtraArgument2=0  MeasurementFcn3=myMeasurementFcn  HasMeasurementJacobianFcn3=off  HasMeasurementEnablePort3=off  HasAdditiveMeasurementNoise3=Additive  MeasurementNoise3=1  HasTimeVaryingMeasurementNoise3=off  HasMeasurementFcnExtraArgument3=0  MeasurementFcn4=myMeasurementFcn  HasMeasurementJacobianFcn4=off  HasMeasurementEnablePort4=off  HasAdditiveMeasurementNoise4=Additive  MeasurementNoise4=1  HasTimeVaryingMeasurementNoise4=off  HasMeasurementFcnExtraArgument4=0  MeasurementFcn5=myMeasurementFcn  HasMeasurementJacobianFcn5=off  HasMeasurementEnablePort5=off  HasAdditiveMeasurementNoise5=Additive  MeasurementNoise5=1  HasTimeVaryingMeasurementNoise5=off  HasMeasurementFcnExtraArgument5=0  EnableMultirate=on  StateTransitionFcnSampleTime=SkywalkerX8.Sensors.EKF.GPSSmoothing.StateTransitionSampleTime  MeasurementFcn1SampleTime=SkywalkerX8.Sensors.EKF.GPSSmoothing.MeasurementSampleTime  MeasurementFcn2SampleTime=1  MeasurementFcn3SampleTime=1  MeasurementFcn4SampleTime=1  MeasurementFcn5SampleTime=1  UseCurrentEstimator=on  OutputStateCovariance=off  DataType=double  SampleTime=SkywalkerX8.Sensors.EKF.GPSSmoothing.SampleTime  NumberOfMeasurements=1
      settings: SourceProductName=Control System Toolbox  SourceProductBaseCode=CT
  Gain : Gain  Gain=SkywalkerX8.Sensors.GPS.Velocity.StdDev
  Math Function1 : Math  Operator=magnitude^2  SaturateOnIntegerOverflow=on
  Mux : Mux  Inputs=2
  Mux1 : Mux  Inputs=7
  Overwrite Chi Variance : dspmtrx3/Overwrite Values  OverWriteDiag=Submatrix  valFrom2ndIP=Second input port  ConstValue=0  RowSpan=One row  RowStartMode=Index  RowStartIndex=4  RowEndMode=Last  RowEndIndex=1  ColSpan=One column  ColStartMode=First  ColStartIndex=1  ColEndMode=Last  ColEndIndex=1  DiagSpan=Range of elements  DiagStartMode=Index  DiagStartIndex=2  DiagEndMode=Index  DiagEndIndex=4
      settings: SourceProductName=DSP System Toolbox  SourceProductBaseCode=DS
  Rate Transition : RateTransition  InitialCondition=SkywalkerX8.Sensors.EKF.GPSSmoothing.InitialInput  OutPortSampleTime=SkywalkerX8.Sensors.EKF.GPSSmoothing.StateTransitionSampleTime
  Rate Transition1 : RateTransition  InitialCondition=SkywalkerX8.Sensors.EKF.GPSSmoothing.InitialInput  OutPortSampleTime=SkywalkerX8.Sensors.EKF.GPSSmoothing.MeasurementSampleTime
  Rate Transition2 : RateTransition  InitialCondition=SkywalkerX8.Sensors.EKF.GPSSmoothing.InitialMeasurement  OutPortSampleTime=SkywalkerX8.Sensors.EKF.GPSSmoothing.MeasurementSampleTime
  Reciprocal : MATLAB Function  TreatAsAtomicUnit=on
  Selector : Selector  InputPortWidth=7  IndexOptions=Index vector (dialog)  Indices=3  OutputSizes=1
  Unit Delay : UnitDelay  InitialCondition=SkywalkerX8.Sensors.EKF.GPSSmoothing.InitialState(3)  SampleTime=SkywalkerX8.Sensors.EKF.GPSSmoothing.MeasurementSampleTime
  xhat : Outport
  wires:
  y/1 -> Rate Transition2/1
  GPS Smoothing Extended Kalman Filter/1 -> Demux3/1, Selector/1
  Reciprocal/1(y) -> Gain/1  "1/Vg"
  Gain/1 -> Math Function1/1  "sigma_V/Vg"
  Math Function1/1 -> Overwrite Chi Variance/2  "Chi_var"
  Constant/1 -> Overwrite Chi Variance/1
  Overwrite Chi Variance/1 -> GPS Smoothing Extended Kalman Filter/3
  u/1 -> Rate Transition1/1, Rate Transition/1
  Selector/1 -> Unit Delay/1  "Vg"
  Unit Delay/1 -> Reciprocal/1(u)
  Rate Transition1/1 -> GPS Smoothing Extended Kalman Filter/4
  Rate Transition2/1 -> GPS Smoothing Extended Kalman Filter/2
  Rate Transition/1 -> Mux/1
  Mux/1 -> GPS Smoothing Extended Kalman Filter/1
  Constant1/1 -> Mux/2
  Demux3/1 -> Mux1/1
  Demux3/2 -> Mux1/2
  Demux3/3 -> Mux1/3
  Mux1/1 -> xhat/1
  Demux3/4 -> Chi Low Pass Filter/1
  Chi Low Pass Filter/1 -> Mux1/4
  Demux3/5 -> Mux1/5
  Demux3/6 -> Mux1/6
  Demux3/7 -> Mux1/7

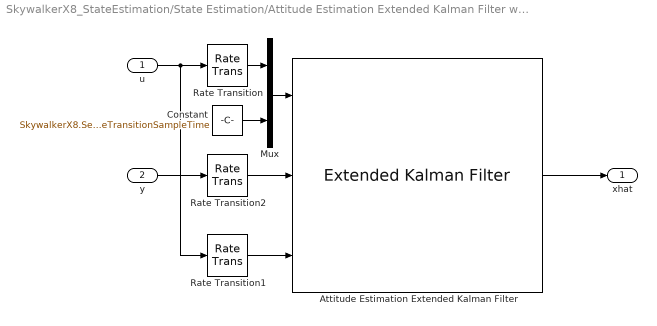
== system SkywalkerX8_StateEstimation/State Estimation/Attitude Estimation Extended Kalman Filter with Filtering/Attitude Estimation Extended Kalman Filter ==
  u : Inport
  y : Inport  Port=2
  Attitude Estimation Extended Kalman Filter : sharedTrackingLibrary/Extended Kalman Filter  StateTransitionFcn=attitudeTransitionEstimate  HasStateTransitionJacobianFcn=on  StateTransitionJacobianFcn=attitudeTransitionEstimate_Jacobian  HasAdditiveProcessNoise=Additive  ProcessNoise=SkywalkerX8.Sensors.EKF.Attitude.ProcessCovarianceMatrix  HasTimeVaryingProcessNoise=off  HasStateTransitionFcnExtraArgument=1  InitialState=SkywalkerX8.Sensors.EKF.Attitude.InitialState  InitialStateCovariance=SkywalkerX8.Sensors.EKF.Attitude.InitialStateCovarianceMatrix  MeasurementFcn1=accelerometerMeasurementEstimate  HasMeasurementJacobianFcn1=on  MeasurementJacobianFcn1=accelerometerMeasurementEstimate_Jacobian  HasMeasurementEnablePort1=off  HasAdditiveMeasurementNoise1=Additive  MeasurementNoise1=SkywalkerX8.Sensors.EKF.Attitude.MeasurementCovarianceMatrix  HasTimeVaryingMeasurementNoise1=off  HasMeasurementFcnExtraArgument1=1  MeasurementFcn2=myMeasurementFcn  HasMeasurementJacobianFcn2=off  HasMeasurementEnablePort2=off  HasAdditiveMeasurementNoise2=Additive  MeasurementNoise2=1  HasTimeVaryingMeasurementNoise2=off  HasMeasurementFcnExtraArgument2=0  MeasurementFcn3=myMeasurementFcn  HasMeasurementJacobianFcn3=off  HasMeasurementEnablePort3=off  HasAdditiveMeasurementNoise3=Additive  MeasurementNoise3=1  HasTimeVaryingMeasurementNoise3=off  HasMeasurementFcnExtraArgument3=0  MeasurementFcn4=myMeasurementFcn  HasMeasurementJacobianFcn4=off  HasMeasurementEnablePort4=off  HasAdditiveMeasurementNoise4=Additive  MeasurementNoise4=1  HasTimeVaryingMeasurementNoise4=off  HasMeasurementFcnExtraArgument4=0  MeasurementFcn5=myMeasurementFcn  HasMeasurementJacobianFcn5=off  HasMeasurementEnablePort5=off  HasAdditiveMeasurementNoise5=Additive  MeasurementNoise5=1  HasTimeVaryingMeasurementNoise5=off  HasMeasurementFcnExtraArgument5=0  EnableMultirate=on  StateTransitionFcnSampleTime=SkywalkerX8.Sensors.EKF.Attitude.StateTransitionSampleTime  MeasurementFcn1SampleTime=SkywalkerX8.Sensors.EKF.Attitude.MeasurementSampleTime  MeasurementFcn2SampleTime=1  MeasurementFcn3SampleTime=1  MeasurementFcn4SampleTime=1  MeasurementFcn5SampleTime=1  UseCurrentEstimator=on  OutputStateCovariance=off  DataType=double  SampleTime=SkywalkerX8.Sensors.EKF.Attitude.StateTransitionSampleTime  NumberOfMeasurements=1
      settings: SourceProductName=Control System Toolbox  SourceProductBaseCode=CT
  Constant : Constant  Value=SkywalkerX8.Sensors.EKF.Attitude.StateTransitionSampleTime
  Mux : Mux  Inputs=2
  Rate Transition : RateTransition  InitialCondition=SkywalkerX8.Sensors.EKF.Attitude.InitialInput  OutPortSampleTime=SkywalkerX8.Sensors.EKF.Attitude.StateTransitionSampleTime
  Rate Transition1 : RateTransition  InitialCondition=SkywalkerX8.Sensors.EKF.Attitude.InitialInput  OutPortSampleTime=SkywalkerX8.Sensors.EKF.Attitude.MeasurementSampleTime
  Rate Transition2 : RateTransition  InitialCondition=SkywalkerX8.Sensors.EKF.Attitude.InitialMeasurement  OutPortSampleTime=SkywalkerX8.Sensors.EKF.Attitude.MeasurementSampleTime
  xhat : Outport
  wires:
  y/1 -> Rate Transition2/1
  u/1 -> Rate Transition1/1, Rate Transition/1
  Attitude Estimation Extended Kalman Filter/1 -> xhat/1
  Rate Transition1/1 -> Attitude Estimation Extended Kalman Filter/3
  Rate Transition2/1 -> Attitude Estimation Extended Kalman Filter/2
  Mux/1 -> Attitude Estimation Extended Kalman Filter/1
  Rate Transition/1 -> Mux/1
  Constant/1 -> Mux/2

== matlab function SkywalkerX8_StateEstimation/State Estimation/GPS Smoothing Extended Kalman Filter/Reciprocal ==
  data: u input; y output
function y = reciprocal(u)

    if (u ~= 0)
       y = 1/u;
    else
       y = 1E06; 
    end

end
